simulink model "Taller6"  (R2024a)
settings: Solver=VariableStepAuto  StartTime=0.0  StopTime=20  RelTol=1e-3
settings Model: Creator=emili  LastModifiedBy=emili

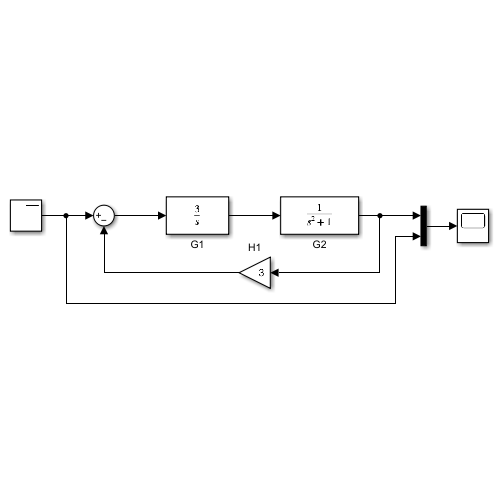
[thumbnail: Simulink's stored preview of the top-level diagram]
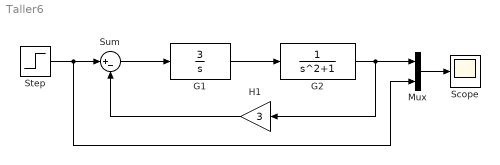
== system Taller6 ==
  G1 : TransferFcn  Numerator=3  Denominator=[1 0]
  G2 : TransferFcn  Numerator=1  Denominator=[1 0 1]
  H1 : Gain  Gain=3
  Mux : Mux  Inputs=2
  Scope : Scope
  Step : Step  After=10  SampleTime=0
  Sum : Sum  Inputs=|+-
  wires:
  Step/1 -> Mux/2, Sum/1
  Sum/1 -> G1/1
  G1/1 -> G2/1
  G2/1 -> Mux/1, H1/1
  H1/1 -> Sum/2
  Mux/1 -> Scope/1
